simulink model "sltankrule"  (Simulink 7.3)
settings: Solver=ode45  SolverMode=SingleTasking  StartTime=0  StopTime=Inf  MaxStep=0.2  RelTol=1e-3  AbsTol=1e-6
PreLoadFcn:
  | tank=readfis('tank');
undefined symbols (not defined in the file or in its folder): D, I, InitialPosition, lb, ub, xi
libraries: fuzblock x1
Description:
  | Water Level Control in a Tank
  | 
  | This demo shows how to use a fuzzy-logic inference system in a Simulink(R) model.
  | 
  | There are two inputs to the fuzzy controller: the rate of change of the water level and
  | the difference between the actual and the required water levels. The controller uses
  | these inputs to control the inflow rate.
  | 
  | When you run the model, the Rule Viewer updates dynamically to show which rule
  | the fuzzy controller is using to set the flow rate.
CloseFcn:
  | AnimFigH = findobj(0,'Name', 'Tank Demo'); close(AnimFigH),ruleFigH = findobj(0,'Name', 'Rule Viewer: tank'); close(ruleFigH)
settings Model: Creator=pascal  LastModifiedBy=matthew
settings DataIOCC: LimitDataPoints=off  SaveOutput=off  SaveTime=off
settings OptimizationCC: BlockReduction=off  BooleanDataType=off  InitFltsAndDblsToZero=on  EfficientMapNaN2IntZero=off
settings DebuggingCC: SaveWithParameterizedLinksMsg=none  SignalResolutionControl=TryResolveAllWithWarning  SolverPrmCheckMsg=none  MultiTaskDSMMsg=warning  MultiTaskCondExecSysMsg=none  SigSpecEnsureSampleTimeMsg=none  StrictBusMsg=None
settings HardwareCC: TargetUnknown=on
settings RTWCC: TemplateMakefile=grt_unix.tmf  IncludeERTFirstTime=on
settings GRTTargetCC: TargetFcnLib=ansi_tfl_tmw.mat

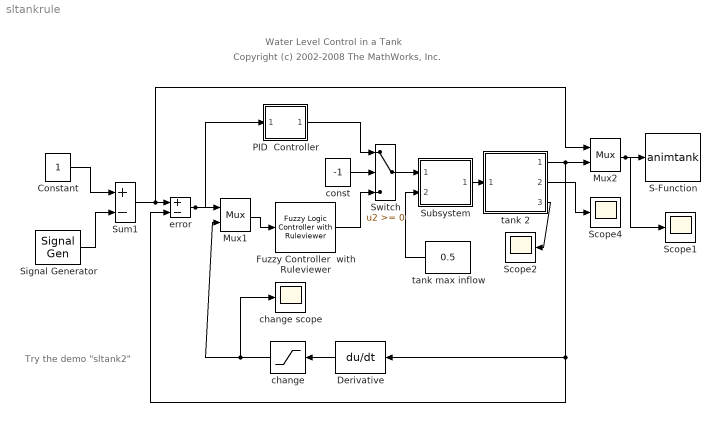
== system sltankrule ==
  note: Try the demo
      | "sltank2"
  note: Water Level Control in a Tank
  note: Copyright (c) 2002-2008 The MathWorks, Inc.
  Constant : Constant  OutDataType=sfix(16)  OutScaling=2^0
  Derivative : Derivative  Orientation=left
  Fuzzy Controller  with Ruleviewer : fuzblock/Fuzzy Logic  Controller  with Ruleviewer  SystemSampleTime=-1  fismatrix=tank  Ts=2
  Mux1 : Mux  Inputs=2
  Mux2 : Mux  Inputs=2
  PID  Controller : Subsystem  mask(PID Controller){P=2,  I=0,  D=1}
      mask prompts: P "Proportional:";  I "Integral";  D "Derivative:"
      mask help:
      | Enter expressions for proportional, integral, and derivative terms.
      | P+I/s+Ds
      mask Help: This block implements a PID controller where parameters are entered for the Proportional, Integral and Derivative terms. Unmask this block to see how it works. The derivative term is implemented using a true derivative block.
      mask Display: disp('PID')
  S-Function : S-Function  FunctionName=animtank  Parameters=1  EnableBusSupport=off
  Scope1 : Scope
      settings: TickLabels=on  TimeRange=200.000000  YMin=-2.000000  YMax=2.000000  DataFormat=Array
  Scope2 : Scope
      settings: TickLabels=on  TimeRange=20.000000  YMin=-2.000000  YMax=2.000000  DataFormat=Array
  Scope4 : Scope
      settings: TickLabels=on  TimeRange=200.000000  YMin=-2.000000  YMax=2.000000  DataFormat=Array
  Signal Generator : SignalGenerator  WaveForm=square  Amplitude=0.500000  Frequency=0.100000  Units=rad/sec
  Subsystem : Subsystem  mask(Valve){InitialPosition =0}
      mask prompts: InitialPosition  "Initial position [0=closed 1=open]:"
      mask help: Valve
      mask Display: disp('VALVE')
  Sum1 : Sum  Inputs=+-  OutDataType=sfix(16)  OutScaling=2^0  SaturateOnIntegerOverflow=on  InputSameDT=on  OutDataTypeStr=Inherit: Same as first input
  Switch : Switch  SaturateOnIntegerOverflow=on  InputSameDT=on
  change : Saturate  Orientation=left  UpperLimit=0.1  LowerLimit=-0.1
  change scope : Scope
      settings: TickLabels=on  TimeRange=20.000000  YMin=-0.100000  YMax=0.100000  DataFormat=Array
  const : Constant  Value=-1  OutDataType=sfix(16)  OutScaling=2^0
  error : Sum  Inputs=+-  OutDataType=sfix(16)  OutScaling=2^0  SaturateOnIntegerOverflow=on  InputSameDT=on  OutDataTypeStr=Inherit: Same as first input
  tank 2 : Subsystem  mask(Water tank){ht=2, area=1, outletArea=0.05, overflowLimit=0, initialHt=0.5}
      mask prompts: ht "Height of tank (m):"; area "Bottom area (m^2):"; outletArea "Out pipe crossection (m^2):"; overflowLimit "Overflow sensor distance from top (m):"; initialHt "Initial level height (m):"
      mask help: Cylindrical water tank with overflow signal
      mask Display: disp('WATER\nTANK')
  tank max inflow : Constant  Orientation=left  Value=0.5  OutDataType=sfix(16)  OutScaling=2^0
  wires:
  tank 2/2(flow out) -> Scope4/1
  tank max inflow/1 -> Subsystem/2(source flow)
  Derivative/1 -> change/1
  Mux1/1 -> Fuzzy Controller  with Ruleviewer/1
  change/1 -> Mux1/2, change scope/1
  Constant/1 -> Sum1/1
  Signal Generator/1 -> Sum1/2
  Subsystem/1(out flow) -> tank 2/1(flow in)
  tank 2/1(water level) -> Mux2/2, error/2, Derivative/1
  Sum1/1 -> error/1, Mux2/1
  tank 2/3(overflow flag) -> Scope2/1
  Switch/1 -> Subsystem/1(control)
  Mux2/1 -> S-Function/1, Scope1/1
  error/1 -> Mux1/1, PID  Controller/1(In_1)
  Fuzzy Controller  with Ruleviewer/1 -> Switch/3
  PID  Controller/1(Out_1) -> Switch/1
  const/1 -> Switch/2

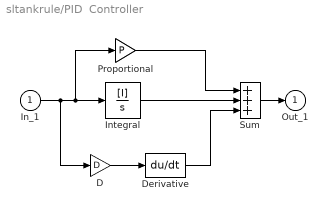
== system sltankrule/PID  Controller ==
  In_1 : Inport  OutDataType=sfix(16)  OutScaling=2^0
  D : Gain  Gain=D  ParameterDataType=sfix(16)  ParameterScaling=2^0  OutDataType=sfix(16)  OutScaling=2^0  SaturateOnIntegerOverflow=on  OutDataTypeStr=Inherit: Same as input  ParamDataTypeStr=Inherit: Same as input
  Derivative : Derivative
  Integral : TransferFcn  Numerator=[I]  Denominator=[1 0]
  Proportional : Gain  Gain=P  ParameterDataType=sfix(16)  ParameterScaling=2^0  OutDataType=sfix(16)  OutScaling=2^0  SaturateOnIntegerOverflow=on  OutDataTypeStr=Inherit: Same as input  ParamDataTypeStr=Inherit: Same as input
  Sum : Sum  Inputs=+++  OutDataType=sfix(16)  OutScaling=2^0  SaturateOnIntegerOverflow=on  InputSameDT=on  OutDataTypeStr=Inherit: Same as first input
  Out_1 : Outport  OutDataType=sfix(16)  OutScaling=2^0  InitialOutput=0
  wires:
  Proportional/1 -> Sum/1
  Integral/1 -> Sum/2
  Derivative/1 -> Sum/3
  In_1/1 -> Integral/1, Proportional/1, D/1
  Sum/1 -> Out_1/1
  D/1 -> Derivative/1

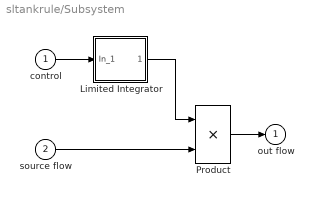
== system sltankrule/Subsystem ==
  control : Inport  OutDataType=sfix(16)  OutScaling=2^0
  source flow : Inport  Port=2  OutDataType=sfix(16)  OutScaling=2^0
  Limited Integrator : Subsystem  mask(Limited integrator.){lb =0,  ub =1,  xi =InitialPosition}
      mask prompts: lb  "Lower bound:";  ub  "Upper bound:";  xi  "Initial condition"
      mask help: Limited integrator
      mask Help: Implements a limited integrator with \nan expression of the form:\n\nif(x<=lb and u<0) or (x>=ub and u>0)\n\txdot=0\nelse\n\txdot=u.
      mask Display: plot(-1,-0.2,3.5,1.2,[0.05,1,2,2.9],[0,0,1,1]);disp(' 1/s    ')
  Product : Product  OutDataType=sfix(16)  OutScaling=2^0  SaturateOnIntegerOverflow=on  RndMeth=Zero  InputSameDT=on  OutDataTypeStr=Inherit: Same as first input
  out flow : Outport  OutDataType=sfix(16)  OutScaling=2^0  InitialOutput=0
  wires:
  source flow/1 -> Product/2
  Product/1 -> out flow/1
  control/1 -> Limited Integrator/1(In_1)
  Limited Integrator/1(Out_1) -> Product/1

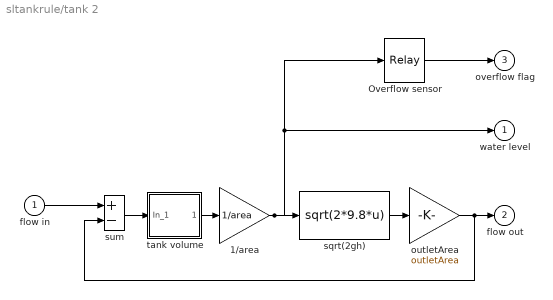
== system sltankrule/tank 2 ==
  flow in : Inport  OutDataType=sfix(16)  OutScaling=2^0
  1/area : Gain  Gain=1/area  ParameterDataType=sfix(16)  ParameterScaling=2^0  OutDataType=sfix(16)  OutScaling=2^0  SaturateOnIntegerOverflow=on  OutDataTypeStr=Inherit: Same as input  ParamDataTypeStr=Inherit: Same as input
  Overflow sensor : Relay  OnSwitchValue=ht - overflowLimit  OffSwitchValue=ht - overflowLimit  OutDataType=sfix(16)  OutScaling=2^0
  outletArea : Gain  Gain=outletArea  ParameterDataType=sfix(16)  ParameterScaling=2^0  OutDataType=sfix(16)  OutScaling=2^0  SaturateOnIntegerOverflow=on  OutDataTypeStr=Inherit: Same as input  ParamDataTypeStr=Inherit: Same as input
  sqrt(2gh) : Fcn  Expr=sqrt(2*9.8*u)
  sum : Sum  Inputs=+-  OutDataType=sfix(16)  OutScaling=2^0  SaturateOnIntegerOverflow=on  InputSameDT=on  OutDataTypeStr=Inherit: Same as first input
  tank volume : Subsystem  mask(Limited integrator.){lb =0,  ub =ht * area,  xi =initialHt * area}
      mask prompts: lb  "Lower bound:";  ub  "Upper bound:";  xi  "Initial condition"
      mask help: Limited integrator
      mask Help: Implements a limited integrator with \nan expression of the form:\n\nif(x<=lb and u<0) or (x>=ub and u>0)\n\txdot=0\nelse\n\txdot=u.
      mask Display: plot(-1,-0.2,3.5,1.2,[0.05,1,2,2.9],[0,0,1,1]);disp(' 1/s    ')
  water level : Outport  OutDataType=sfix(16)  OutScaling=2^0  InitialOutput=0
  flow out : Outport  Port=2  OutDataType=sfix(16)  OutScaling=2^0  InitialOutput=0
  overflow flag : Outport  Port=3  OutDataType=sfix(16)  OutScaling=2^0  InitialOutput=0
  wires:
  outletArea/1 -> flow out/1, sum/2
  sqrt(2gh)/1 -> outletArea/1
  1/area/1 -> Overflow sensor/1, water level/1, sqrt(2gh)/1
  tank volume/1(Out_1) -> 1/area/1
  Overflow sensor/1 -> overflow flag/1
  flow in/1 -> sum/1
  sum/1 -> tank volume/1(In_1)

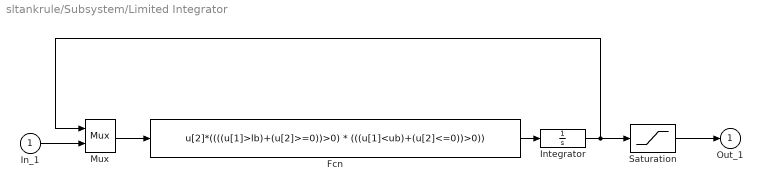
== system sltankrule/Subsystem/Limited Integrator ==
  In_1 : Inport  OutDataType=sfix(16)  OutScaling=2^0
  Fcn : Fcn  Expr=u[2]*((((u[1]>lb)+(u[2]>=0))>0) * (((u[1]<ub)+(u[2]<=0))>0))
  Integrator : Integrator  InitialCondition=xi
  Mux : Mux  Inputs=2
  Saturation : Saturate  UpperLimit=ub  LowerLimit=lb
  Out_1 : Outport  OutDataType=sfix(16)  OutScaling=2^0  InitialOutput=0
  wires:
  Integrator/1 -> Saturation/1, Mux/1
  Fcn/1 -> Integrator/1
  Mux/1 -> Fcn/1
  In_1/1 -> Mux/2
  Saturation/1 -> Out_1/1

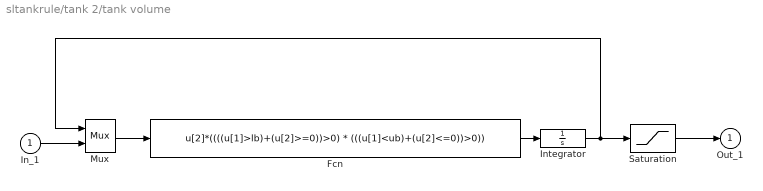
== system sltankrule/tank 2/tank volume ==
  In_1 : Inport  OutDataType=sfix(16)  OutScaling=2^0
  Fcn : Fcn  Expr=u[2]*((((u[1]>lb)+(u[2]>=0))>0) * (((u[1]<ub)+(u[2]<=0))>0))
  Integrator : Integrator  InitialCondition=xi
  Mux : Mux  Inputs=2
  Saturation : Saturate  UpperLimit=ub  LowerLimit=lb
  Out_1 : Outport  OutDataType=sfix(16)  OutScaling=2^0  InitialOutput=0
  wires:
  Integrator/1 -> Saturation/1, Mux/1
  Fcn/1 -> Integrator/1
  Mux/1 -> Fcn/1
  In_1/1 -> Mux/2
  Saturation/1 -> Out_1/1
